simulink subsystem "Speed_PI_C"  (R2022b)
settings: Solver=VariableStepAuto  StartTime=0.0  StopTime=10.0  RelTol=1e-3
undefined symbols (not defined in the file or in its folder): conv, motor, Ri, Rw, sat
settings Model: Creator=gotta  LastModifiedBy=gotta

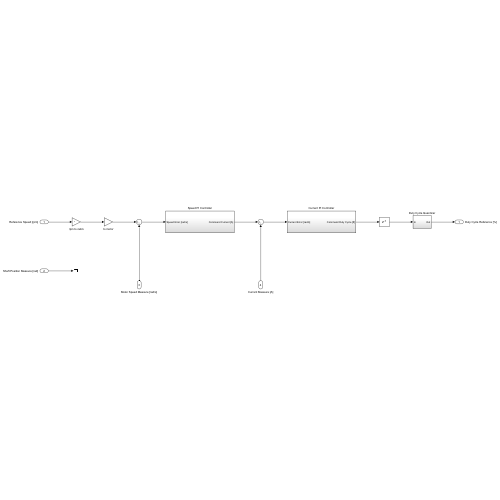
[thumbnail: Simulink's stored preview of the top-level diagram]
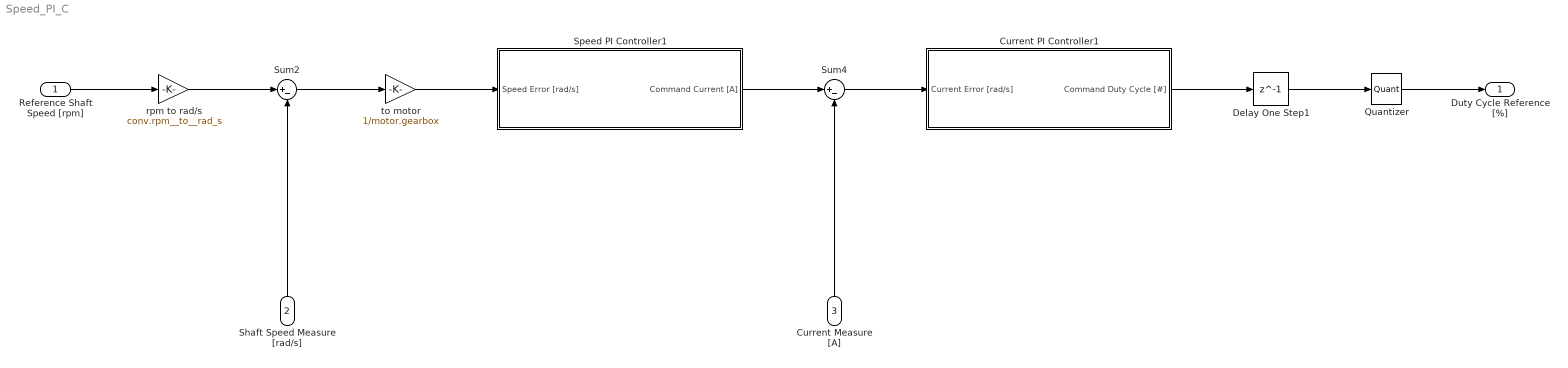
== system Speed_PI_C ==
  Reference Shaft Speed [rpm] : Inport
  Shaft Speed Measure [rad/s] : Inport  Port=2
  Current Measure [A] : Inport  Port=3
  Current PI Controller1 : Subsystem
  Delay One Step1 : Delay  DelayLength=1
  Quantizer : Quantizer  QuantizationInterval=uc.duty_step
  Speed PI Controller1 : Subsystem
  Sum2 : Sum  Inputs=|+-
  Sum4 : Sum  Inputs=|+-
  rpm to rad/s : Gain  Gain=conv.rpm__to__rad_s
  to motor : Gain  Gain=1/motor.gearbox
  Duty Cycle Reference [%] : Outport
  wires:
  Delay One Step1/1 -> Quantizer/1
  Quantizer/1 -> Duty Cycle Reference [%]/1
  Sum2/1 -> to motor/1
  Current PI Controller1/1(Command Duty Cycle [#]) -> Delay One Step1/1
  Sum4/1 -> Current PI Controller1/1(Current Error [rad/s])
  Current Measure [A]/1 -> Sum4/2
  Shaft Speed Measure [rad/s]/1 -> Sum2/2
  rpm to rad/s/1 -> Sum2/1
  Speed PI Controller1/1(Command Current [A]) -> Sum4/1
  Reference Shaft Speed [rpm]/1 -> rpm to rad/s/1
  to motor/1 -> Speed PI Controller1/1(Speed Error [rad/s])

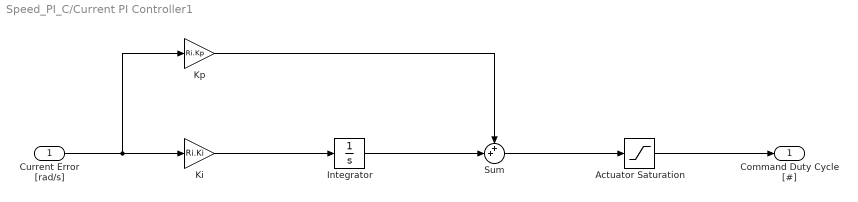
== system Speed_PI_C/Current PI Controller1 ==
  Current Error [rad/s] : Inport
  Actuator Saturation : Saturate  UpperLimit=sat.d  LowerLimit=-sat.d
  Integrator : Integrator  LimitOutput=on  UpperSaturationLimit=sat.d  LowerSaturationLimit=-sat.d
  Ki : Gain  Gain=Ri.Ki
  Kp : Gain  Gain=Ri.Kp
  Sum : Sum  Inputs=++|
  Command Duty Cycle [#] : Outport
  wires:
  Integrator/1 -> Sum/2
  Ki/1 -> Integrator/1
  Sum/1 -> Actuator Saturation/1
  Kp/1 -> Sum/1
  Current Error [rad/s]/1 -> Ki/1, Kp/1
  Actuator Saturation/1 -> Command Duty Cycle [#]/1

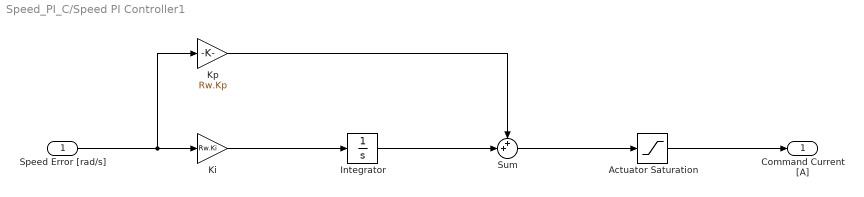
== system Speed_PI_C/Speed PI Controller1 ==
  Speed Error [rad/s] : Inport
  Actuator Saturation : Saturate  UpperLimit=sat.I  LowerLimit=-sat.I
  Integrator : Integrator  LimitOutput=on  UpperSaturationLimit=sat.I  LowerSaturationLimit=-sat.I
  Ki : Gain  Gain=Rw.Ki
  Kp : Gain  Gain=Rw.Kp
  Sum : Sum  Inputs=++|
  Command Current [A] : Outport
  wires:
  Integrator/1 -> Sum/2
  Ki/1 -> Integrator/1
  Sum/1 -> Actuator Saturation/1
  Speed Error [rad/s]/1 -> Kp/1, Ki/1
  Actuator Saturation/1 -> Command Current [A]/1
  Kp/1 -> Sum/1
